simulink model "lamp_heater"  (R2024a)
settings: Solver=FixedStepDiscrete  StartTime=0.0  StopTime=inf  FixedStep=0.1  RelTol=1e-3
libraries: etargetslib x6, instrumentseriallib x3
settings Model: Creator=setm  LastModifiedBy=setm

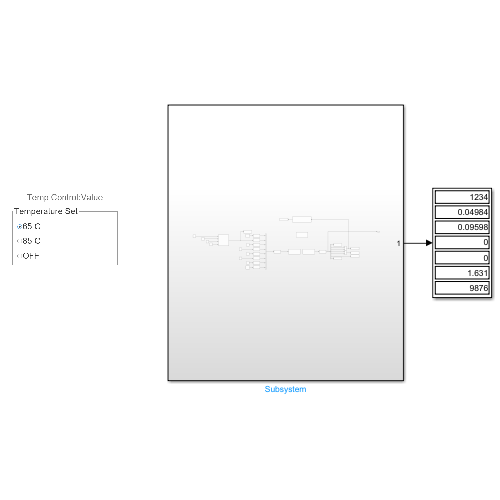
[thumbnail: Simulink's stored preview of the top-level diagram]
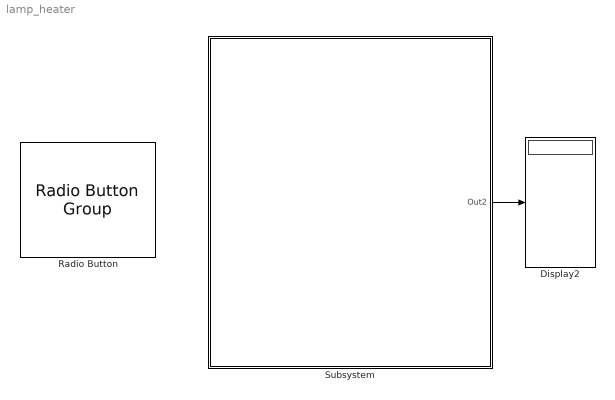
== system lamp_heater ==
  Display2 : Display
      settings: Decimation=5
  Radio Button : RadioButtonGroup  SelectedLabel=65 C  ButtonGroupName=Temperature Set
      settings: Values={{'65 C', '85 C', 'OFF'}, [0 1 2]}
  Subsystem : Subsystem
  wires:
  Subsystem/1(Out2) -> Display2/1

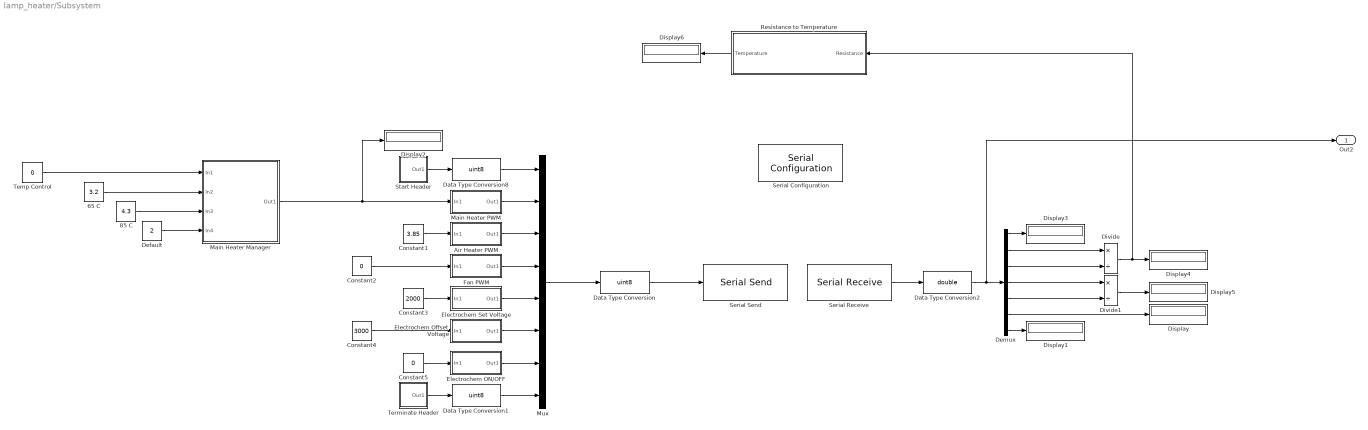
== system lamp_heater/Subsystem ==
  65 C : Constant  Value=3.2
  85 C : Constant  Value=4.3
  Air Heater PWM : Subsystem
  Constant1 : Constant  Value=3.85
  Constant2 : Constant  Value=0
  Constant3 : Constant  Value=2000
  Constant4 : Constant  Value=3000
  Constant5 : Constant  Value=0
  Data Type Conversion : DataTypeConversion  OutDataTypeStr=uint8  SaturateOnIntegerOverflow=off  RndMeth=Floor
  Data Type Conversion1 : DataTypeConversion  OutDataTypeStr=uint8  SaturateOnIntegerOverflow=off  RndMeth=Floor
  Data Type Conversion2 : DataTypeConversion  OutDataTypeStr=double  SaturateOnIntegerOverflow=off  RndMeth=Floor
  Data Type Conversion8 : DataTypeConversion  OutDataTypeStr=uint8  SaturateOnIntegerOverflow=off  RndMeth=Floor
  Default : Constant  Value=2
  Demux : Demux  Outputs=7
  Display{,1..6} (7 alike) : Display
      Display1 settings: Decimation=5
      Display3 settings: Decimation=5
  Divide : Product  Inputs=*/
  Divide1 : Product  Inputs=*/
  Electrochem ON/OFF : Subsystem
  Electrochem Offset Voltage : Subsystem
  Electrochem Set Voltage : Subsystem
  Fan PWM : Subsystem
  Main Heater Manager : Subsystem
  Main Heater PWM : Subsystem
  Mux : Mux  Inputs=8
  Resistance to Temperature : Subsystem
  Serial Configuration : instrumentseriallib/Serial Configuration  Priority=-200000  PortSel=COM5  Port=COM5  ComPort=COM5  BaudRate=115200  DataBits=8  Parity=none  StopBits=1  ByteOrder=little-endian  FlowControl=none  Timeout=10  SimulateUsing=Interpreted execution  BlockInModel=on  aMode=1
  Serial Receive : instrumentseriallib/Serial Receive  Priority=1  PortSel=COM5  Port=COM5  ComPort=COM5  DataType=single  SaveDataType=uint8  ToggleHeader=off  Header=[]  ToggleDataSize=on  DataSize=[7 1]  ToggleTerminator=off  Terminator=<none>  CustomTerminator=[]  InputFormat=Column major  EnableBlockingMode=on  ActionDataUnavailable=Output last received value  ActionWhenDataUnavailable=Output last received value  CustomValue=0  SampleTime=0.1  SimulateUsing=Interpreted execution  BlockInModel=on  aMode=1
  Serial Send : instrumentseriallib/Serial Send  Priority=1  PortSel=COM5  Port=COM5  ComPort=COM5  Header=[]  Terminator=<none>  CustomTerminator=[]  EnableBlockingMode=on  SimulateUsing=Interpreted execution  BlockInModel=on  aMode=1
  Start Header : Subsystem
  Temp Control : Constant  Value=0
  Terminate Header : Subsystem
  Out2 : Outport
  wires:
  Electrochem ON/OFF/1(Out1) -> Mux/7
  Constant2/1 -> Fan PWM/1(In1)
  Divide1/1 -> Display5/1
  Demux/7 -> Display1/1
  Demux/4 -> Divide1/1
  Demux/5 -> Divide1/2
  Mux/1 -> Data Type Conversion/1
  Data Type Conversion1/1 -> Mux/8
  Data Type Conversion8/1 -> Mux/1
  Data Type Conversion/1 -> Serial Send/1
  Air Heater PWM/1(Out1) -> Mux/3
  Constant4/1 -> Electrochem Offset Voltage/1(In1)
  Demux/6 -> Display/1
  Constant1/1 -> Air Heater PWM/1(In1)
  Electrochem Offset Voltage/1(Out1) -> Mux/6
  Constant3/1 -> Electrochem Set Voltage/1(In1)
  Demux/3 -> Divide/2
  Serial Receive/1 -> Data Type Conversion2/1
  Constant5/1 -> Electrochem ON/OFF/1(In1)
  Fan PWM/1(Out1) -> Mux/4
  Divide/1 -> Resistance to Temperature/1(Resistance), Display4/1
  Electrochem Set Voltage/1(Out1) -> Mux/5
  Main Heater PWM/1(Out1) -> Mux/2
  Demux/2 -> Divide/1
  Start Header/1(Out1) -> Data Type Conversion8/1
  Resistance to Temperature/1(Temperature) -> Display6/1
  Demux/1 -> Display3/1
  Terminate Header/1(Out1) -> Data Type Conversion1/1
  Data Type Conversion2/1 -> Out2/1, Demux/1
  Main Heater Manager/1(Out1) -> Display2/1, Main Heater PWM/1(In1)
  65 C/1 -> Main Heater Manager/2(In2)
  Default/1 -> Main Heater Manager/4(In4)
  85 C/1 -> Main Heater Manager/3(In3)
  Temp Control/1 -> Main Heater Manager/1(In1)

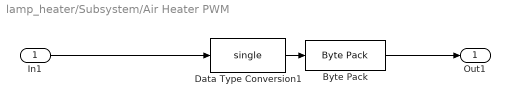
== system lamp_heater/Subsystem/Air Heater PWM ==
  In1 : Inport
  Byte Pack : etargetslib/Byte Pack  datatypes={'single'}  byteAlign=1
  Data Type Conversion1 : DataTypeConversion  OutDataTypeStr=single  SaturateOnIntegerOverflow=off  RndMeth=Floor
  Out1 : Outport
  wires:
  Data Type Conversion1/1 -> Byte Pack/1
  Byte Pack/1 -> Out1/1
  In1/1 -> Data Type Conversion1/1

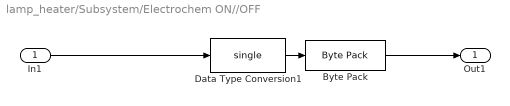
== system lamp_heater/Subsystem/Electrochem ON//OFF ==
  In1 : Inport
  Byte Pack : etargetslib/Byte Pack  datatypes={'single'}  byteAlign=1
  Data Type Conversion1 : DataTypeConversion  OutDataTypeStr=single  SaturateOnIntegerOverflow=off  RndMeth=Floor
  Out1 : Outport
  wires:
  Data Type Conversion1/1 -> Byte Pack/1
  Byte Pack/1 -> Out1/1
  In1/1 -> Data Type Conversion1/1

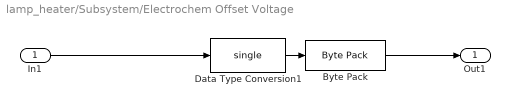
== system lamp_heater/Subsystem/Electrochem Offset Voltage ==
  In1 : Inport
  Byte Pack : etargetslib/Byte Pack  datatypes={'single'}  byteAlign=1
  Data Type Conversion1 : DataTypeConversion  OutDataTypeStr=single  SaturateOnIntegerOverflow=off  RndMeth=Floor
  Out1 : Outport
  wires:
  Data Type Conversion1/1 -> Byte Pack/1
  Byte Pack/1 -> Out1/1
  In1/1 -> Data Type Conversion1/1

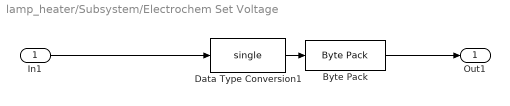
== system lamp_heater/Subsystem/Electrochem Set Voltage ==
  In1 : Inport
  Byte Pack : etargetslib/Byte Pack  datatypes={'single'}  byteAlign=1
  Data Type Conversion1 : DataTypeConversion  OutDataTypeStr=single  SaturateOnIntegerOverflow=off  RndMeth=Floor
  Out1 : Outport
  wires:
  Data Type Conversion1/1 -> Byte Pack/1
  Byte Pack/1 -> Out1/1
  In1/1 -> Data Type Conversion1/1

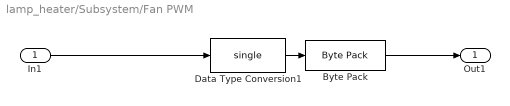
== system lamp_heater/Subsystem/Fan PWM ==
  In1 : Inport
  Byte Pack : etargetslib/Byte Pack  datatypes={'single'}  byteAlign=1
  Data Type Conversion1 : DataTypeConversion  OutDataTypeStr=single  SaturateOnIntegerOverflow=off  RndMeth=Floor
  Out1 : Outport
  wires:
  Data Type Conversion1/1 -> Byte Pack/1
  Byte Pack/1 -> Out1/1
  In1/1 -> Data Type Conversion1/1

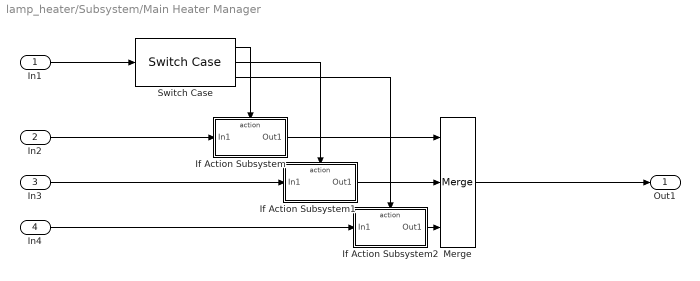
== system lamp_heater/Subsystem/Main Heater Manager ==
  In1 : Inport
  In2 : Inport  Port=2
  In3 : Inport  Port=3
  In4 : Inport  Port=4
  If Action Subsystem : Subsystem  TreatAsAtomicUnit=on
  If Action Subsystem1 : Subsystem  TreatAsAtomicUnit=on
  If Action Subsystem2 : Subsystem  TreatAsAtomicUnit=on
  Merge : Merge  Inputs=3  InitialOutput=[0]
  Switch Case : SwitchCase  CaseConditions={0, 1}
  Out1 : Outport
  wires:
  Switch Case/2 -> If Action Subsystem1/Action
  If Action Subsystem/1(Out1) -> Merge/1
  Merge/1 -> Out1/1
  Switch Case/1 -> If Action Subsystem/Action
  If Action Subsystem1/1(Out1) -> Merge/2
  Switch Case/3 -> If Action Subsystem2/Action
  In1/1 -> Switch Case/1
  If Action Subsystem2/1(Out1) -> Merge/3
  In2/1 -> If Action Subsystem/1(In1)
  In3/1 -> If Action Subsystem1/1(In1)
  In4/1 -> If Action Subsystem2/1(In1)

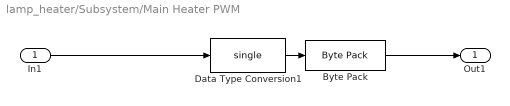
== system lamp_heater/Subsystem/Main Heater PWM ==
  In1 : Inport
  Byte Pack : etargetslib/Byte Pack  datatypes={'single'}  byteAlign=1
  Data Type Conversion1 : DataTypeConversion  OutDataTypeStr=single  SaturateOnIntegerOverflow=off  RndMeth=Floor
  Out1 : Outport
  wires:
  Data Type Conversion1/1 -> Byte Pack/1
  Byte Pack/1 -> Out1/1
  In1/1 -> Data Type Conversion1/1

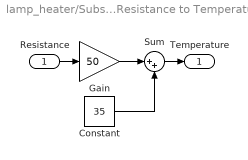
== system lamp_heater/Subsystem/Resistance to Temperature ==
  Resistance : Inport
  Constant : Constant  Value=35
  Gain : Gain  Gain=50
  Sum : Sum  Inputs=|++
  Temperature : Outport
  wires:
  Gain/1 -> Sum/1
  Constant/1 -> Sum/2
  Resistance/1 -> Gain/1
  Sum/1 -> Temperature/1

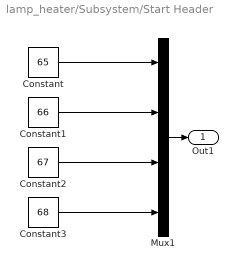
== system lamp_heater/Subsystem/Start Header ==
  Constant : Constant  Value=65
  Constant1 : Constant  Value=66
  Constant2 : Constant  Value=67
  Constant3 : Constant  Value=68
  Mux1 : Mux
  Out1 : Outport
  wires:
  Constant/1 -> Mux1/1
  Constant3/1 -> Mux1/4
  Constant2/1 -> Mux1/3
  Constant1/1 -> Mux1/2
  Mux1/1 -> Out1/1

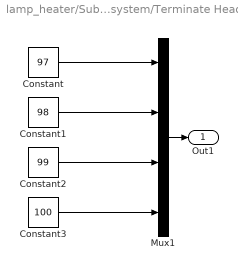
== system lamp_heater/Subsystem/Terminate Header ==
  Constant : Constant  Value=97
  Constant1 : Constant  Value=98
  Constant2 : Constant  Value=99
  Constant3 : Constant  Value=100
  Mux1 : Mux
  Out1 : Outport
  wires:
  Constant/1 -> Mux1/1
  Constant3/1 -> Mux1/4
  Constant2/1 -> Mux1/3
  Constant1/1 -> Mux1/2
  Mux1/1 -> Out1/1

== system lamp_heater/Subsystem/Main Heater Manager/If Action Subsystem ==
  In1 : Inport
  Action Port : ActionPort  ActionPortLabel=case [ 0 ]:
  Out1 : Outport
  wires:
  In1/1 -> Out1/1

== system lamp_heater/Subsystem/Main Heater Manager/If Action Subsystem1 ==
  In1 : Inport
  Action Port : ActionPort  ActionPortLabel=case [ 1 ]:
  Out1 : Outport
  wires:
  In1/1 -> Out1/1

== system lamp_heater/Subsystem/Main Heater Manager/If Action Subsystem2 ==
  In1 : Inport
  Action Port : ActionPort  ActionPortLabel=default:
  Out1 : Outport
  wires:
  In1/1 -> Out1/1
